simulink subsystem "Nonlinear_Plant"  (R2020b)
settings: Solver=VariableStepAuto  StartTime=0.0  StopTime=10.0  RelTol=1e-3
undefined symbols (not defined in the file): Earth, inertia, initial, mass, WGS84
libraries: sharedtransform x2, sharedutil x2, aerolibtransform2 x1
settings Model: Creator=Fatih  LastModifiedBy=Fatih

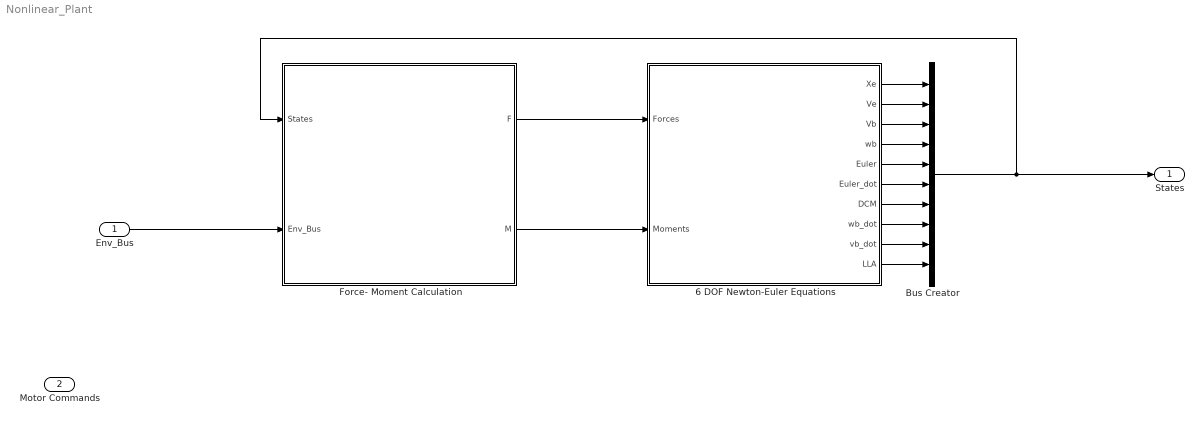
== system Nonlinear_Plant ==
  Env_Bus : Inport
  Motor Commands : Inport  Port=2
  "6 DOF Newton-Euler Equations " : Subsystem
  Bus Creator : BusCreator  Inputs=10
  Force- Moment Calculation : Subsystem
  States : Outport
  wires:
  "6 DOF Newton-Euler Equations "/8(wb_dot) -> Bus Creator/8
  "6 DOF Newton-Euler Equations "/6(Euler_dot) -> Bus Creator/6
  "6 DOF Newton-Euler Equations "/10("LLA ") -> Bus Creator/10
  "6 DOF Newton-Euler Equations "/7(DCM) -> Bus Creator/7
  "6 DOF Newton-Euler Equations "/2(Ve) -> Bus Creator/2
  "6 DOF Newton-Euler Equations "/9(vb_dot) -> Bus Creator/9
  "6 DOF Newton-Euler Equations "/4(wb) -> Bus Creator/4
  "6 DOF Newton-Euler Equations "/1(Xe) -> Bus Creator/1
  "6 DOF Newton-Euler Equations "/5(Euler) -> Bus Creator/5
  "6 DOF Newton-Euler Equations "/3(Vb) -> Bus Creator/3
  Bus Creator/1 -> States/1, Force- Moment Calculation/1(States)
  Force- Moment Calculation/1(F) -> "6 DOF Newton-Euler Equations "/1("Forces ")
  Force- Moment Calculation/2(M) -> "6 DOF Newton-Euler Equations "/2(Moments)
  Env_Bus/1 -> Force- Moment Calculation/2(Env_Bus)

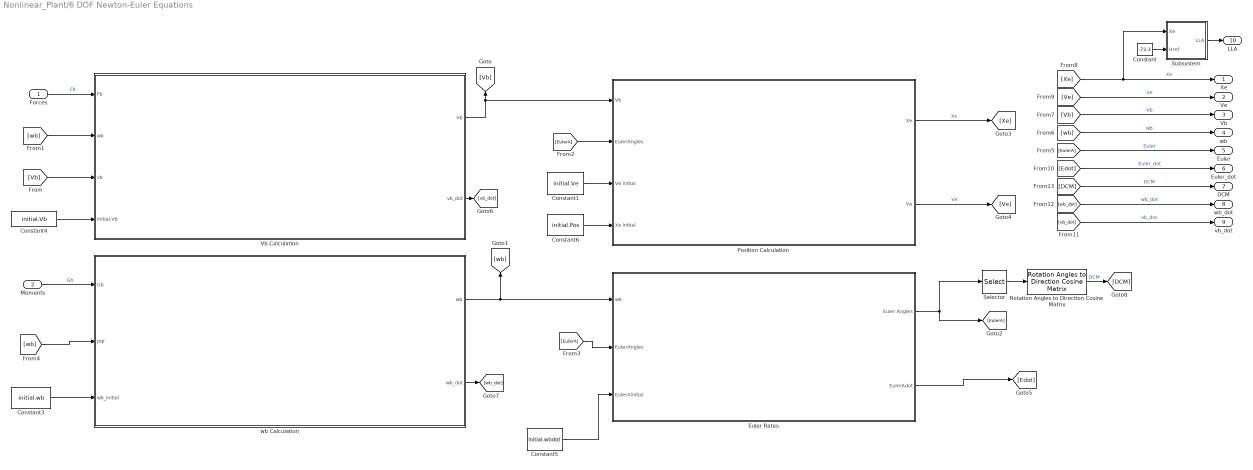
== system Nonlinear_Plant/6 DOF Newton-Euler Equations  ==
  "Forces " : Inport
  Moments : Inport  Port=2
  Constant : Constant  Value=-72.3
  Constant1 : Constant  Value=initial.Ve
  Constant3 : Constant  Value=initial.wb
  Constant4 : Constant  Value=initial.Vb
  Constant5 : Constant  Value=initial.wbdot
  Constant6 : Constant  Value=initial.Pos
  Euler Rates : Subsystem
  "Position Calculation " : Subsystem
  Rotation Angles to Direction Cosine Matrix : sharedtransform/Rotation Angles to Direction Cosine Matrix  rotationOrder=ZYX  aMode=aMode
      settings: SourceProductBaseCode=AE,PW,MT,VE,VP
  Selector : Selector  InputPortWidth=3  IndexOptions=Index vector (dialog)  Indices=[3 2 1]  OutputSizes=1
  Subsystem : Subsystem
  Vb Calculation : Subsystem
  wb Calculation : Subsystem
  Xe : Outport
  Ve : Outport  Port=2
  Vb : Outport  Port=3
  wb : Outport  Port=4
  Euler : Outport  Port=5
  Euler_dot : Outport  Port=6
  DCM : Outport  Port=7
  wb_dot : Outport  Port=8
  vb_dot : Outport  Port=9
  "LLA " : Outport  Port=10
  wires:
  Subsystem/1(LLA) -> "LLA "/1
  Constant/1 -> Subsystem/2(Href)
  [DCM] -> DCM/1  "DCM"
  Rotation Angles to Direction Cosine Matrix/1 -> [DCM]  "DCM"
  [Xe] -> Xe/1, Subsystem/1(Xe)  "Xe"
  [Ve] -> Ve/1  "Ve"
  [Vb] -> Vb/1  "Vb"
  [wb] -> wb/1  "wb"
  [EulerA] -> Euler/1  "Euler"
  [Edot] -> Euler_dot/1  "Euler_dot"
  [wb_dot] -> wb_dot/1  "wb_dot"
  [vb_dot] -> vb_dot/1  "vb_dot"
  wb Calculation/2("wb_dot ") -> [wb_dot]
  Vb Calculation/2(vb_dot) -> [vb_dot]
  Euler Rates/2("EulerAdot ") -> [Edot]
  Selector/1 -> Rotation Angles to Direction Cosine Matrix/1
  Constant1/1 -> "Position Calculation "/3("Ve initial ")
  Constant6/1 -> "Position Calculation "/4("Xe initial ")
  "Position Calculation "/2(Ve) -> [Ve]  "Ve"
  "Position Calculation "/1(Xe) -> [Xe]  "Xe"
  Moments/1 -> wb Calculation/1(Gb)  "Gb"
  [EulerA] -> "Position Calculation "/2(EulerAngles)
  Euler Rates/1(Euler Angles) -> [EulerA], Selector/1
  Constant5/1 -> Euler Rates/3("EulerAinitial ")
  [EulerA] -> Euler Rates/2(EulerAngles)
  Constant3/1 -> wb Calculation/3("wb_initial ")
  [wb] -> wb Calculation/2(pqr)
  wb Calculation/1(wb) -> Euler Rates/1(wb), [wb]
  Constant4/1 -> Vb Calculation/4(initial.Vb)
  [Vb] -> Vb Calculation/3("vb ")
  [wb] -> Vb Calculation/2(wb)
  "Forces "/1 -> Vb Calculation/1(Fb)  "Fb"
  Vb Calculation/1(Vb) -> "Position Calculation "/1(Vb), [Vb]

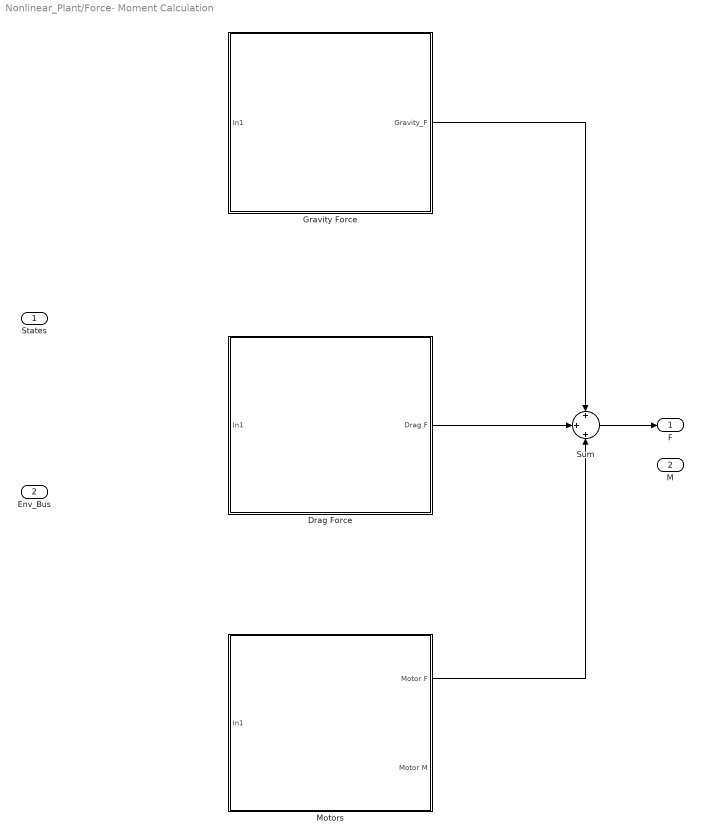
== system Nonlinear_Plant/Force- Moment Calculation ==
  States : Inport
  Env_Bus : Inport  Port=2
  Drag Force : Subsystem
  Gravity Force : Subsystem
  Motors : Subsystem
  Sum : Sum  Inputs=+|+|+
  F : Outport
  M : Outport  Port=2
  wires:
  Sum/1 -> F/1
  Motors/1(Motor F) -> Sum/3
  Gravity Force/1(Gravity_F) -> Sum/1
  Drag Force/1(Drag F) -> Sum/2

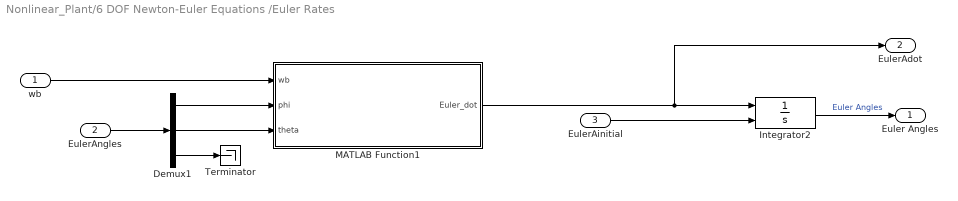
== system Nonlinear_Plant/6 DOF Newton-Euler Equations /Euler Rates ==
  wb : Inport
  EulerAngles : Inport  Port=2
  "EulerAinitial " : Inport  Port=3
  Demux1 : Demux  Outputs=3
  Integrator2 : Integrator  InitialConditionSource=external  LimitOutput=on  UpperSaturationLimit=[pi; pi/2;pi]  LowerSaturationLimit=[-pi;-pi/2 ;-pi]  WrappedStateUpperValue=[pi; pi/2;pi]  WrappedStateLowerValue=[-pi;-pi/2 ;-pi]  IgnoreLimit=on
  MATLAB Function1 : MATLAB Function  TreatAsAtomicUnit=on
  Terminator : Terminator
  Euler Angles : Outport
  "EulerAdot " : Outport  Port=2
  wires:
  MATLAB Function1/1(Euler_dot) -> "EulerAdot "/1, Integrator2/1
  EulerAngles/1 -> Demux1/1
  "EulerAinitial "/1 -> Integrator2/2
  wb/1 -> MATLAB Function1/1(wb)
  Demux1/1 -> MATLAB Function1/2(phi)
  Demux1/2 -> MATLAB Function1/3(theta)
  Integrator2/1 -> Euler Angles/1  "Euler Angles"
  Demux1/3 -> Terminator/1

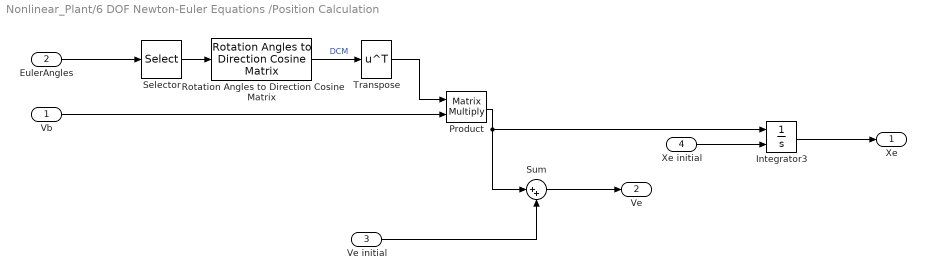
== system Nonlinear_Plant/6 DOF Newton-Euler Equations /Position Calculation  ==
  Vb : Inport
  EulerAngles : Inport  Port=2
  "Ve initial " : Inport  Port=3
  "Xe initial " : Inport  Port=4
  Integrator3 : Integrator  InitialConditionSource=external
  Product : Product  Multiplication=Matrix(*)
  Rotation Angles to Direction Cosine Matrix : sharedtransform/Rotation Angles to Direction Cosine Matrix  rotationOrder=ZYX  aMode=aMode
      settings: SourceProductBaseCode=AE,PW,MT,VE,VP
  Selector : Selector  InputPortWidth=3  IndexOptions=Index vector (dialog)  Indices=[3 2 1]  OutputSizes=1
  Sum : Sum  Inputs=|++
  Transpose : Math  Operator=transpose  SaturateOnIntegerOverflow=on
  Xe : Outport
  Ve : Outport  Port=2
  wires:
  Vb/1 -> Product/2
  Transpose/1 -> Product/1
  Rotation Angles to Direction Cosine Matrix/1 -> Transpose/1  "DCM"
  Selector/1 -> Rotation Angles to Direction Cosine Matrix/1
  "Ve initial "/1 -> Sum/2
  Sum/1 -> Ve/1
  Integrator3/1 -> Xe/1
  "Xe initial "/1 -> Integrator3/2
  EulerAngles/1 -> Selector/1
  Product/1 -> Integrator3/1, Sum/1

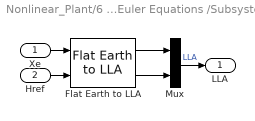
== system Nonlinear_Plant/6 DOF Newton-Euler Equations /Subsystem ==
  Xe : Inport
  Href : Inport  Port=2
  Flat Earth to LLA : aerolibtransform2/Flat Earth to LLA  units=Metric (MKS)  ptype=Earth (WGS84)  F=1/298.257223563  R=6378137  LL0=[0 10]  psi=0
  Mux : Mux  Inputs=2
  LLA : Outport
  wires:
  Mux/1 -> LLA/1  "LLA"
  Flat Earth to LLA/2 -> Mux/2
  Flat Earth to LLA/1 -> Mux/1
  Href/1 -> Flat Earth to LLA/2
  Xe/1 -> Flat Earth to LLA/1

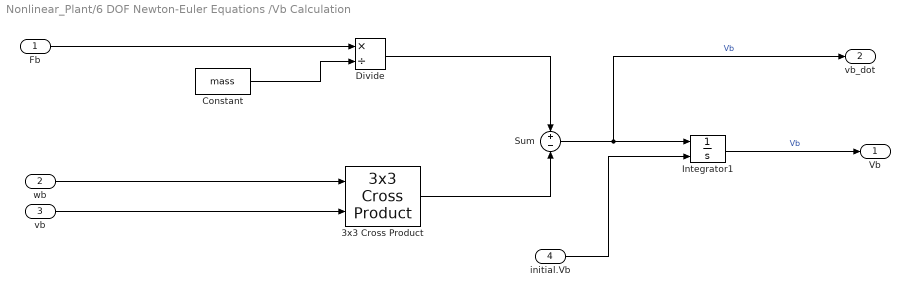
== system Nonlinear_Plant/6 DOF Newton-Euler Equations /Vb Calculation ==
  Fb : Inport
  wb : Inport  Port=2
  "vb " : Inport  Port=3
  initial.Vb : Inport  Port=4
  3x3 Cross Product : sharedutil/3x3 Cross Product  aMode=aMode
      settings: SourceProductBaseCode=AE,PW,MT,VE,VP
  Constant : Constant  Value=mass
  Divide : Product  Inputs=*/
  Integrator1 : Integrator  InitialConditionSource=external
  Sum : Sum  Inputs=+|-
  Vb : Outport
  vb_dot : Outport  Port=2
  wires:
  initial.Vb/1 -> Integrator1/2
  Sum/1 -> Integrator1/1, vb_dot/1  "Vb"
  "vb "/1 -> 3x3 Cross Product/2
  Integrator1/1 -> Vb/1  "Vb"
  Divide/1 -> Sum/1
  Constant/1 -> Divide/2
  Fb/1 -> Divide/1
  wb/1 -> 3x3 Cross Product/1
  3x3 Cross Product/1 -> Sum/2

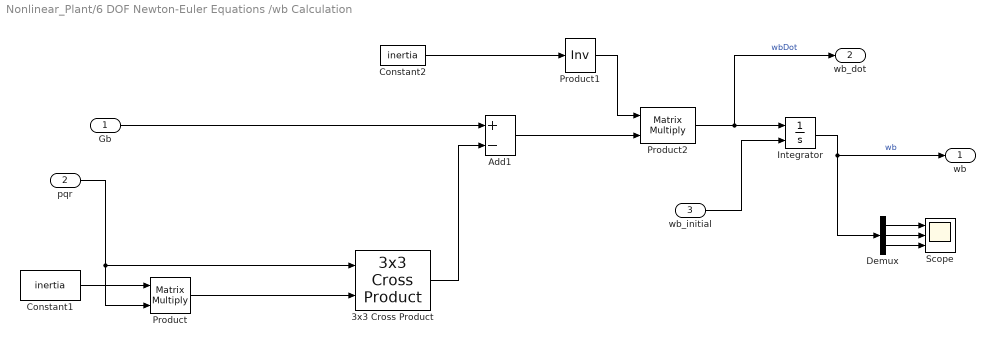
== system Nonlinear_Plant/6 DOF Newton-Euler Equations /wb Calculation ==
  Gb : Inport
  pqr : Inport  Port=2
  "wb_initial " : Inport  Port=3
  3x3 Cross Product : sharedutil/3x3 Cross Product  aMode=aMode
      settings: SourceProductBaseCode=AE,PW,MT,VE,VP
  Add1 : Sum  Inputs=+-
  Constant1 : Constant  Value=inertia
  Constant2 : Constant  Value=inertia
  Demux : Demux  Outputs=3
  Integrator : Integrator  InitialConditionSource=external
  Product : Product  Multiplication=Matrix(*)
  Product1 : Product  Inputs=/  Multiplication=Matrix(*)
  Product2 : Product  Multiplication=Matrix(*)
  Scope : Scope  NumInputPorts=3
  wb : Outport
  "wb_dot " : Outport  Port=2
  wires:
  Product/1 -> 3x3 Cross Product/2
  pqr/1 -> 3x3 Cross Product/1, Product/2
  Constant1/1 -> Product/1
  Product1/1 -> Product2/1
  Product2/1 -> "wb_dot "/1, Integrator/1  "wbDot"
  Constant2/1 -> Product1/1
  Demux/3 -> Scope/3
  Demux/2 -> Scope/2
  Demux/1 -> Scope/1
  Gb/1 -> Add1/1
  Integrator/1 -> Demux/1, wb/1  "wb"
  3x3 Cross Product/1 -> Add1/2
  Add1/1 -> Product2/2
  "wb_initial "/1 -> Integrator/2

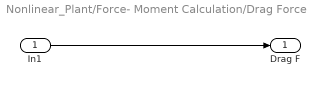
== system Nonlinear_Plant/Force- Moment Calculation/Drag Force ==
  In1 : Inport
  Drag F : Outport
  wires:
  In1/1 -> Drag F/1

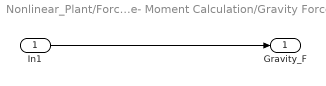
== system Nonlinear_Plant/Force- Moment Calculation/Gravity Force ==
  In1 : Inport
  Gravity_F : Outport
  wires:
  In1/1 -> Gravity_F/1

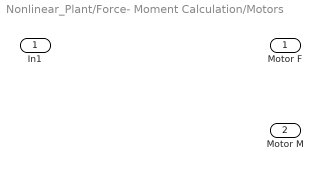
== system Nonlinear_Plant/Force- Moment Calculation/Motors ==
  In1 : Inport
  Motor F : Outport
  Motor M : Outport  Port=2

== matlab function Nonlinear_Plant/6 DOF Newton-Euler Equations /Euler Rates/MATLAB Function1 ==
  data: wb input; phi input; theta input; Euler_dot output
function Euler_dot = EulerRates(wb,phi,theta)

RMatrix = [1 0 -sin(theta);...
    0 cos(phi) sin(phi)*cos(theta);...
    0 -sin(phi) cos(phi)*cos(theta)];

Euler_dot = inv(RMatrix) * wb;
end
